simulink model " PV_PEM_reconfigurable_battery"  (R2026a)
settings: Solver=VariableStepAuto  StopTime=sim_t
undefined symbols (not defined in the file or in its folder): Active_Area, Bi_L, N, Q_batt, Ra_stack, Rc_stack, Rint_stack, sample_output_time, SOC_max, SOC_min, THR_75_down, THR_75_up, THR_97_down, THR_97_up, Ts, V_ref_battery, Vint_stack
libraries: fl_lib x30, nesl_utility x22, ee_lib x5, simulink x4, batteryecm_lib x1, slpidlib x1
settings Model: Creator=hanna  LastModifiedBy=Diamantis
settings SimscapeCC: SimscapeNominalValues="[{\"value\":\"1\",\"unit\":\"A\"},{\"value\":\"1\",\"unit\":\"bar\"},{\"value\":\"1\",\"unit\":\"cm^2\"},{\"value\":\"1\",\"unit\":\"cm^3/s\"},{\"value\":\"1\",\"unit\":\"kJ/kg\"},{\"value\":\"1\",\"unit\":\"kW\"},{\"value\":\"1\",\"unit\":\"l\"},{\"value\":\"1\",\"unit\":\"N\"},{\"value\":\"1\",\"unit\":\"N*m\"},{\"value\":\"1\",\"unit\":\"V\"}]"  SimscapeLogType=none  SimscapeLogDataHistory=5000.0

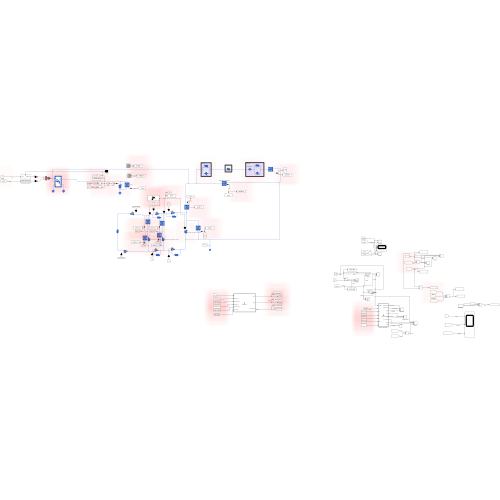
[thumbnail: Simulink's stored preview of the top-level diagram]
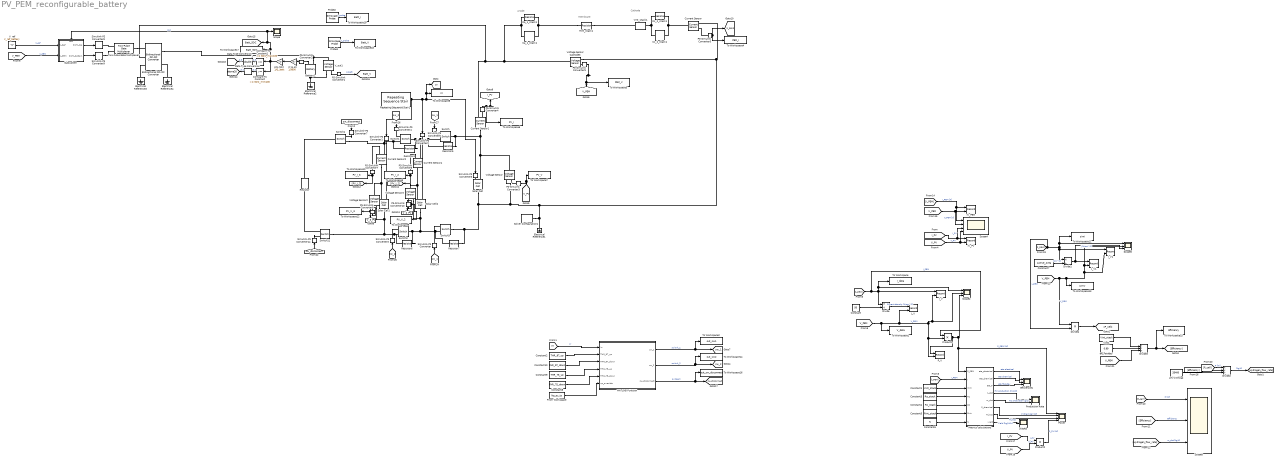
== system  PV_PEM_reconfigurable_battery ==
  note: Membrane
  note: Cathode
  note: Anode
  Battery1 : batteryecm_lib/Battery  Vnom=V_batt_nom V  prm_dir=simscape.enum.battery.prm_dir.disabled  R1_dis=0.05 Ohm  R1_ch=0.05 Ohm  R1=0.01 Ohm  prm_AH=simscape.enum.battery.prm_AH.finite  AH=Q_batt A*hr  V1=11.5 V  AH1=Q_batt*(SOC_min/100) A*hr  prm_R2=simscape.enum.battery.prm_R2.disabled  R2=2000 Ohm  Tmeas=298.15 K  charge_measurement_port=simscape.enum.battery.enable.yes  prm_dyn=simscape.enum.battery.prm_dyn.off  Rp1=0.005 Ohm  tau1=30 s  Rp2=0.005 Ohm  tau2=30 s  Rp3=0.005 Ohm  tau3=30 s  Rp4=0.005 Ohm  tau4=30 s  Rp5=0.005 Ohm  tau5=30 s  prm_fade=simscape.enum.battery.prm_fade.disabled  N_fade=100  AH_fade=45 A*hr  R1_fade=2.02 Ohm  R1_ch_fade=2.02 Ohm  V1_fade=10.35 V  prm_age=simscape.enum.battery.prm_age.disabled  prm_age_OCV=simscape.enum.battery.prm_age_OCV.OCV  OCV_age=0.9  SOC_age=60  Tmeas_age=298.15 K  delta_time_age_vec=[0] d  temperature_age_vec=[273] K  OCV_scaling_age=2.2134e6  OCV_offset_age=1.632e6  temp_exp_age=0.515833569 V  t_exp_age=0.75  Vnom_T2=12 V  R1_T2=2.2 Ohm  R1_T2_dis=2.2 Ohm  R1_T2_ch=2.2 Ohm  V1_T2=11.4 V  R2_T2=2200 Ohm  Rp1_T2=0.005 Ohm  tau1_T2=30 s  Rp2_T2=0.005 Ohm  tau2_T2=30 s  Rp3_T2=0.005 Ohm  tau3_T2=30 s  Rp4_T2=0.005 Ohm  tau4_T2=30 s  Rp5_T2=0.005 Ohm  tau5_T2=30 s  Tmeas2=273.15 K  thermal_port=simscape.enum.thermaleffects.omit  thermal_mass=30000 J/K  i_specify=off  i_priority=None  i=0 A  i_nominal_specify=off  i_nominal_value=1  i_nominal_unit=A  v_specify=off  v_priority=None  v=0 V  v_nominal_specify=off  v_nominal_value=1  v_nominal_unit=V  charge_specify=on  charge_priority=High  charge=SOC_init A*hr  charge_nominal_specify=off  charge_nominal_value=1  charge_nominal_unit=A*hr  num_cycles_specify=off  num_cycles_priority=High  num_cycles=0  num_cycles_nominal_specify=off  num_cycles_nominal_value=1  num_cycles_nominal_unit=1  temperature_specify=off  temperature_priority=High  temperature=298.15 K  temperature_nominal_specify=off  temperature_nominal_value=1  temperature_nominal_unit=K
      settings: LibrarySourceBlock=batt_lib/Cells/Battery
  Bidirectional DC-DC Converter : ee_lib/Semiconductors & Converters/Converters/Bidirectional DC-DC Converter  fidelity_option=ee.enum.converters.fidelity.detailed  device_type=ee.enum.converters.switchingdevice.mosfet  Vf=0.8 V  Ron=0.001 Ohm  Rds=0.001 Ohm  Goff=1e-6 1/Ohm  Vth=2 V  Vgt=0.5 V  Vgt_off=-1 V  Ih=1 A  K=0  diode_param=ee.enum.converters.diode.nodynamics  diode_Vf=0.8 V  diode_Ron=0.001 Ohm  diode_Goff=1e-5 1/Ohm  diode_C=50 nF  diode_iRM=-5 A  diode_iF=50 A  diode_idot=-50 A/us  diode_trr_param=ee.enum.converters.diodetrr.trr_factor  diode_trr_factor=3  diode_trr=0.5 us  diode_Qrr=1500 s*uA  L=Bi_L H  Rl=0 Ohm  C1=Bi_C1 F  C2=Bi_C2 F  R1=Bi_R1 Ohm  R2=Bi_R2 Ohm  snubber_type=ee.enum.converters.snubber.exclude  Cs=1e-7 F  Rs=0.1 Ohm  iL_specify=off  iL_priority=High  iL=0 A  iL_nominal_specify=off  iL_nominal_value=1  iL_nominal_unit=A  vc1_specify=off  vc1_priority=High  vc1=0 V  vc1_nominal_specify=off  vc1_nominal_value=1  vc1_nominal_unit=V  vc2_specify=off  vc2_priority=High  vc2=0 V  vc2_nominal_specify=off  vc2_nominal_value=1  vc2_nominal_unit=V  device_type_hv=ee.enum.converters.switchingdevice.ideal  Vf_hv=0.8 V  Ron_hv=0.001 Ohm  Rds_hv=0.001 Ohm  Goff_hv=1e-5 1/Ohm  Vth_hv=0.5 V  Vgt_hv=0.5 V  Vgt_off_hv=-1 V  Ih_hv=1 A  device_type_lv=ee.enum.converters.switchingdevice.ideal  Vf_lv=0.8 V  Ron_lv=0.001 Ohm  Rds_lv=0.001 Ohm  Goff_lv=1e-5 1/Ohm  Vth_lv=0.5 V  Vgt_lv=0.5 V  Vgt_off_lv=-1 V  Ih_lv=1 A  T_L1=0.03 H  T_L2=0.03 H  T_k=0.9  snubber_type_hv=ee.enum.converters.snubber.exclude  Cs_hv=1e-7 F  Rs_hv=0.1 Ohm  snubber_type_lv=ee.enum.converters.snubber.exclude  Cs_lv=1e-7 F  Rs_lv=0.1 Ohm  iL1_specify=off  iL1_priority=High  iL1=0 A  iL1_nominal_specify=off  iL1_nominal_value=1  iL1_nominal_unit=A  iL2_specify=off  iL2_priority=High  iL2=0 A  iL2_nominal_specify=off  iL2_nominal_value=1  iL2_nominal_unit=A  hysteresisCurrent=0.01 A
  C to Ah : Gain  Gain=1/3600
  Ca_1_stack1 : fl_lib/Electrical/Electrical Elements/Capacitor  c=Ca_stack F  r=1e-6 Ohm  g=0 1/Ohm  i_specify=off  i_priority=None  i=0 A  i_nominal_specify=off  i_nominal_value=1  i_nominal_unit=A  v_specify=off  v_priority=None  v=0 V  v_nominal_specify=off  v_nominal_value=1  v_nominal_unit=V  vc_specify=off  vc_priority=High  vc=0 V  vc_nominal_specify=off  vc_nominal_value=1  vc_nominal_unit=V
  Cc_2_stack1 : fl_lib/Electrical/Electrical Elements/Capacitor  c=Cc_stack F  r=1e-6 Ohm  g=0 1/Ohm  i_specify=off  i_priority=None  i=0 A  i_nominal_specify=off  i_nominal_value=1  i_nominal_unit=A  v_specify=off  v_priority=None  v=0 V  v_nominal_specify=off  v_nominal_value=1  v_nominal_unit=V  vc_specify=off  vc_priority=High  vc=0 V  vc_nominal_specify=off  vc_nominal_value=1  vc_nominal_unit=V
  Compare To Constant : simulink/Logic and Bit Operations/Compare To Constant  relop=>=  const=SOC_min/100  OutDataTypeStr=boolean
  Compare To Constant1 : simulink/Logic and Bit Operations/Compare To Constant  relop=<=  const=SOC_max/100  OutDataTypeStr=boolean
  Constant : Constant  Value=50
  Constant1 : Constant  Value=Vint_stack
  Constant10 : Constant  Value=THR_97_down
  Constant2 : Constant  Value=THR_97_up
  Constant3 : Constant  Value=Ra_stack
  Constant4 : Constant  Value=Rc_stack
  Constant5 : Constant  Value=Rint_stack
  Constant6 : Constant  Value=N
  Constant7 : Constant  Value=Active_Area
  Constant8 : Constant  Value=THR_75_down
  Constant9 : Constant  Value=THR_75_up
  Current Sensor{,1..2,4} (4 alike) : fl_lib/Electrical/Electrical Sensors/Current Sensor
  Data Type Conversion : DataTypeConversion  OutDataTypeStr=double  SaturateOnIntegerOverflow=off  RndMeth=Floor
  Data Type Conversion1 : DataTypeConversion  OutDataTypeStr=double  SaturateOnIntegerOverflow=off  RndMeth=Floor
  Divide : Product  Inputs=*/
  Divide1 : Product  Inputs=*/
  Divide2 : Product  Inputs=**/
  Divide3 : Product  Inputs=**/
  Divide4 : Product  Inputs=**
  Efficiencies : Scope  NumInputPorts=3
      settings: ActiveDisplayYMinimum=-1  ActiveDisplayYMaximum=1  DataLoggingMaxPoints=520000  DataLoggingVariableName=ScopeData5
  Electrical Reference{1..4} (4 alike) : fl_lib/Electrical/Electrical Elements/Electrical Reference
  From Workspace : FromWorkspace  VariableName=Np_py_ts
  IV_PEM : Record  NumPorts=2.0  FileSettingsInternal="{\"entries\":[{\"content\":{\"excelSettings\":{\"content\":{},\"type\":\"Streamout.ExcelSettings\"},\"parquetSettings\":{\"content\":{},\"type\":\"Streamout.ParquetSettings\"}},\"type\":\"Streamout.FileSettingStorage\",\"uuid\":\"\"}],\"packageUris\":[\"http:\\/\\/schema.mathworks.com\\/mf0\\/streamout_blocks\\/R2020a\"],\"version\":\"1.0\"}"  FrameSettings=[0, 0]  Layout=[1 1]  SignalsInternal="{\"entries\":[{\"content\":{\"signals\":[{\"content\":{\"blockPath\":[],\"dimensions\":[1],\"domain\":\"\",\"lineColor\":\"#edb120\",\"lineWidth\":2,\"port\":1,\"signalID\":1,\"signalName\":\"I_PEM [A]\"},\"type\":\"RecordBlkView.Signal\",\"uuid\":\"\"},{\"content\":{\"blockPath\":[],\"dimensions\":[1],\"domain\":\"\",\"lineColor\":\"#7e2f8e\",\"lineWidth\":2,\"port\":2,\"signalID\":2,\"signalName\":\"V_PEM [V]\"},\"type\":\"RecordBlkView.Signal\",\"uuid\":\"\"}]},\"type\":\"RecordBlkView.InputSignals\",\"uuid\":\"\"}],\"packageUris\":[\"http:\\/\\/schema.mathworks.com\\/mf0\\/streamout_blocks\\/R2020a\"],\"version\":\"1.0\"}"  VisualizationBindings="{\"xyplotplugin\":{\"info\":[{\"series\":[],\"subplotID\":1}]}}"  CompatibilityTag=XY
  IV_PV : Record  NumPorts=2.0  FileSettingsInternal="{\"entries\":[{\"content\":{\"excelSettings\":{\"content\":{},\"type\":\"Streamout.ExcelSettings\"},\"parquetSettings\":{\"content\":{},\"type\":\"Streamout.ParquetSettings\"}},\"type\":\"Streamout.FileSettingStorage\",\"uuid\":\"\"}],\"packageUris\":[\"http:\\/\\/schema.mathworks.com\\/mf0\\/streamout_blocks\\/R2020a\"],\"version\":\"1.0\"}"  FrameSettings=[0, 0]  Layout=[1 1]  SignalsInternal="{\"entries\":[{\"content\":{\"signals\":[{\"content\":{\"blockPath\":[],\"dimensions\":[1],\"domain\":\"\",\"lineColor\":\"#a2142f\",\"plots\":[ 1 ],\"port\":1,\"signalID\":1,\"signalName\":\"I_PV\"},\"type\":\"RecordBlkView.Signal\",\"uuid\":\"\"},{\"content\":{\"blockPath\":[],\"dimensions\":[1],\"domain\":\"\",\"lineColor\":\"#139fff\",\"plots\":[ 1 ],\"port\":2,\"signalID\":2,\"signalName\":\"V_PV\"},\"type\":\"RecordBlkView.Signal\",\"uuid\":\"\"}]},\"type\":\"RecordBlkView.InputSignals\",\"uuid\":\"\"}],\"packageUris\":[\"http:\\/\\/schema.mathworks.com\\/mf0\\/streamout_blocks\\/R2020a\"],\"version\":\"1.0\"}"  VisualizationBindings="{\"xyplotplugin\":{\"info\":[{\"series\":[{\"bindingParametersList\":[{\"parameter\":\"X-Axis\",\"signalID\":1,\"signalName\":\"I_PV\"},{\"parameter\":\"Y-Axis\",\"signalID\":2,\"signalName\":\"V_PV\"}],\"seriesID\":0}],\"subplotID\":1}]}}"  CompatibilityTag=XY
  I_V : Record  NumPorts=2.0  FileSettingsInternal="{\"entries\":[{\"content\":{\"excelSettings\":{\"content\":{},\"type\":\"Streamout.ExcelSettings\"},\"parquetSettings\":{\"content\":{},\"type\":\"Streamout.ParquetSettings\"}},\"type\":\"Streamout.FileSettingStorage\",\"uuid\":\"\"}],\"packageUris\":[\"http:\\/\\/schema.mathworks.com\\/mf0\\/streamout_blocks\\/R2020a\"],\"version\":\"1.0\"}"  FrameSettings=[0, 0]  Layout=[1 1]  SignalsInternal="{\"entries\":[{\"content\":{\"signals\":[{\"content\":{\"blockPath\":[],\"dimensions\":[1],\"domain\":\"\",\"lineColor\":\"#a2142f\",\"lineWidth\":2,\"port\":1,\"signalID\":1,\"signalName\":\"I_PEM\"},\"type\":\"RecordBlkView.Signal\",\"uuid\":\"\"},{\"content\":{\"blockPath\":[],\"dimensions\":[1],\"domain\":\"\",\"lineColor\":\"#139fff\",\"lineWidth\":2,\"port\":2,\"signalID\":2,\"signalName\":\"V_PEM\"},\"type\":\"RecordBlkView.Signal\",\"uuid\":\"\"}]},\"type\":\"RecordBlkView.InputSignals\",\"uuid\":\"\"}],\"packageUris\":[\"http:\\/\\/schema.mathworks.com\\/mf0\\/streamout_blocks\\/R2020a\"],\"version\":\"1.0\"}"  VisualizationBindings="{\"xyplotplugin\":{\"info\":[{\"series\":[],\"subplotID\":1}]}}"  CompatibilityTag=XY
  I_V1 : Record  NumPorts=2.0  FileSettingsInternal="{\"entries\":[{\"content\":{\"excelSettings\":{\"content\":{},\"type\":\"Streamout.ExcelSettings\"},\"parquetSettings\":{\"content\":{},\"type\":\"Streamout.ParquetSettings\"}},\"type\":\"Streamout.FileSettingStorage\",\"uuid\":\"\"}],\"packageUris\":[\"http:\\/\\/schema.mathworks.com\\/mf0\\/streamout_blocks\\/R2020a\"],\"version\":\"1.0\"}"  FrameSettings=[0, 0]  Layout=[1 1]  SignalsInternal="{\"entries\":[{\"content\":{\"signals\":[{\"content\":{\"blockPath\":[],\"dimensions\":[1],\"domain\":\"\",\"lineColor\":\"#ff6929\",\"lineWidth\":2,\"port\":1,\"signalID\":1,\"signalName\":\"I_PEM\"},\"type\":\"RecordBlkView.Signal\",\"uuid\":\"\"},{\"content\":{\"blockPath\":[],\"dimensions\":[1],\"domain\":\"\",\"lineColor\":\"#b746ff\",\"lineWidth\":2,\"port\":2,\"signalID\":2,\"signalName\":\"V_PEM\"},\"type\":\"RecordBlkView.Signal\",\"uuid\":\"\"}]},\"type\":\"RecordBlkView.InputSignals\",\"uuid\":\"\"}],\"packageUris\":[\"http:\\/\\/schema.mathworks.com\\/mf0\\/streamout_blocks\\/R2020a\"],\"version\":\"1.0\"}"  VisualizationBindings="{\"xyplotplugin\":{\"info\":[{\"series\":[],\"subplotID\":1}]}}"  CompatibilityTag=XY
  J_V : Record  NumPorts=2.0  FileSettingsInternal="{\"entries\":[{\"content\":{\"excelSettings\":{\"content\":{},\"type\":\"Streamout.ExcelSettings\"},\"parquetSettings\":{\"content\":{},\"type\":\"Streamout.ParquetSettings\"}},\"type\":\"Streamout.FileSettingStorage\",\"uuid\":\"\"}],\"packageUris\":[\"http:\\/\\/schema.mathworks.com\\/mf0\\/streamout_blocks\\/R2020a\"],\"version\":\"1.0\"}"  FrameSettings=[0, 0]  Layout=[1 1]  SignalsInternal="{\"entries\":[{\"content\":{\"signals\":[{\"content\":{\"blockPath\":[],\"dimensions\":[1],\"domain\":\"\",\"lineColor\":\"#64d413\",\"lineWidth\":2,\"port\":1,\"signalID\":1,\"signalName\":\"Current density [A\\/cm^2]\"},\"type\":\"RecordBlkView.Signal\",\"uuid\":\"\"},{\"content\":{\"blockPath\":[],\"dimensions\":[1],\"domain\":\"\",\"lineColor\":\"#ff13a6\",\"lineWidth\":2,\"port\":2,\"signalID\":2,\"signalName\":\"V_PEM\"},\"type\":\"RecordBlkView.Signal\",\"uuid\":\"\"}]},\"type\":\"RecordBlkView.InputSignals\",\"uuid\":\"\"}],\"packageUris\":[\"http:\\/\\/schema.mathworks.com\\/mf0\\/streamout_blocks\\/R2020a\"],\"version\":\"1.0\"}"  VisualizationBindings="{\"xyplotplugin\":{\"info\":[{\"series\":[],\"subplotID\":1}]}}"  CompatibilityTag=XY
  J_V1 : Record  NumPorts=2.0  FileSettingsInternal="{\"entries\":[{\"content\":{\"excelSettings\":{\"content\":{},\"type\":\"Streamout.ExcelSettings\"},\"parquetSettings\":{\"content\":{},\"type\":\"Streamout.ParquetSettings\"}},\"type\":\"Streamout.FileSettingStorage\",\"uuid\":\"\"}],\"packageUris\":[\"http:\\/\\/schema.mathworks.com\\/mf0\\/streamout_blocks\\/R2020a\"],\"version\":\"1.0\"}"  FrameSettings=[0, 0]  Layout=[1 1]  SignalsInternal="{\"entries\":[{\"content\":{\"signals\":[{\"content\":{\"blockPath\":[],\"dimensions\":[1],\"domain\":\"\",\"lineColor\":\"#fe330a\",\"lineWidth\":2,\"port\":1,\"signalID\":1,\"signalName\":\"J [A\\/cm^2]\"},\"type\":\"RecordBlkView.Signal\",\"uuid\":\"\"},{\"content\":{\"blockPath\":[],\"dimensions\":[1],\"domain\":\"\",\"lineColor\":\"#22b573\",\"lineWidth\":2,\"port\":2,\"signalID\":2,\"signalName\":\"V_PEM\"},\"type\":\"RecordBlkView.Signal\",\"uuid\":\"\"}]},\"type\":\"RecordBlkView.InputSignals\",\"uuid\":\"\"}],\"packageUris\":[\"http:\\/\\/schema.mathworks.com\\/mf0\\/streamout_blocks\\/R2020a\"],\"version\":\"1.0\"}"  VisualizationBindings="{\"xyplotplugin\":{\"info\":[{\"series\":[],\"subplotID\":1}]}}"  CompatibilityTag=XY
  LHV [Wh/kg] : Constant  Value=33400
  MATLAB Function : MATLAB Function  TreatAsAtomicUnit=on
  Metrics calculations : MATLAB Function  TreatAsAtomicUnit=on
  PS-Simulink Converter{1..2,5..7,9} (6 alike) : nesl_utility/PS-Simulink Converter  PhysicalDomain=network_engine_domain  SubClassName=ps_output  LeftPortType=input  RightPortType=output  PseudoPeriodic=off  Frequencies=[]  VectorFormat=inherit  Unit=inherit  AffineConversion=off
  PS-Simulink Converter10 : nesl_utility/PS-Simulink Converter  PhysicalDomain=network_engine_domain  SubClassName=ps_output  LeftPortType=input  RightPortType=output  PseudoPeriodic=off  Frequencies=[]  VectorFormat=1-D array  Unit=V  AffineConversion=off
  PS-Simulink Converter3 : nesl_utility/PS-Simulink Converter  PhysicalDomain=network_engine_domain  SubClassName=ps_output  LeftPortType=input  RightPortType=output  PseudoPeriodic=off  Frequencies=[]  VectorFormat=1-D array  Unit=V  AffineConversion=off
  PS-Simulink Converter4 : nesl_utility/PS-Simulink Converter  PhysicalDomain=network_engine_domain  SubClassName=ps_output  LeftPortType=input  RightPortType=output  PseudoPeriodic=off  Frequencies=[]  VectorFormat=1-D array  Unit=A  AffineConversion=off
  PS-Simulink Converter8 : nesl_utility/PS-Simulink Converter  PhysicalDomain=network_engine_domain  SubClassName=ps_output  LeftPortType=input  RightPortType=output  PseudoPeriodic=off  Frequencies=[]  VectorFormat=1-D array  Unit=V  AffineConversion=off
  P_V : Record  NumPorts=2.0  FileSettingsInternal="{\"entries\":[{\"content\":{\"excelSettings\":{\"content\":{},\"type\":\"Streamout.ExcelSettings\"},\"parquetSettings\":{\"content\":{},\"type\":\"Streamout.ParquetSettings\"}},\"type\":\"Streamout.FileSettingStorage\",\"uuid\":\"\"}],\"packageUris\":[\"http:\\/\\/schema.mathworks.com\\/mf0\\/streamout_blocks\\/R2020a\"],\"version\":\"1.0\"}"  FrameSettings=[0, 0]  Layout=[1 1]  SignalsInternal="{\"entries\":[{\"content\":{\"signals\":[{\"content\":{\"blockPath\":[],\"dimensions\":[1],\"domain\":\"\",\"lineColor\":\"#0072bd\",\"lineWidth\":2,\"port\":1,\"signalID\":1,\"signalName\":\"P_PEM [W]\"},\"type\":\"RecordBlkView.Signal\",\"uuid\":\"\"},{\"content\":{\"blockPath\":[],\"dimensions\":[1],\"domain\":\"\",\"lineColor\":\"#d95319\",\"lineWidth\":2,\"port\":2,\"signalID\":2,\"signalName\":\"V_PEM\"},\"type\":\"RecordBlkView.Signal\",\"uuid\":\"\"}]},\"type\":\"RecordBlkView.InputSignals\",\"uuid\":\"\"}],\"packageUris\":[\"http:\\/\\/schema.mathworks.com\\/mf0\\/streamout_blocks\\/R2020a\"],\"version\":\"1.0\"}"  VisualizationBindings="{\"xyplotplugin\":{\"info\":[{\"series\":[],\"subplotID\":1}]}}"  CompatibilityTag=XY
  Power : Scope  NumInputPorts=4
      settings: ActiveDisplayYMinimum=-1  ActiveDisplayYMaximum=1  DataLoggingMaxPoints=520000  DataLoggingVariableName=ScopeData6
  Probe1 : SimscapeProbe  BoundBlock=1128  Variables="{\"i\":{\"Probing\":\"OFF\"},\"n.v\":{\"Probing\":\"OFF\"},\"p.v\":{\"Probing\":\"OFF\"},\"v\":{\"Probing\":\"ON\"}}"
  Probe2 : SimscapeProbe  BoundBlock=1128  Variables="{\"i\":{\"Probing\":\"ON\"}}"
  Product1 : Product
  Product2 : Product
  Production Rate : Scope  NumInputPorts=2
      settings: ActiveDisplayYMinimum=-6.6507662971533038E-5  ActiveDisplayYMaximum=0.00059856896673107221  DataLoggingMaxPoints=520000  DataLoggingVariableName=ScopeData7
  Ra_1_stack1 : fl_lib/Electrical/Electrical Elements/Resistor  R=Ra_stack Ohm  i_specify=off  i_priority=None  i=0 A  i_nominal_specify=off  i_nominal_value=1  i_nominal_unit=A  v_specify=off  v_priority=None  v=0 V  v_nominal_specify=off  v_nominal_value=1  v_nominal_unit=V
  Rc_2_stack1 : fl_lib/Electrical/Electrical Elements/Resistor  R=Rc_stack Ohm  i_specify=off  i_priority=None  i=0 A  i_nominal_specify=off  i_nominal_value=1  i_nominal_unit=A  v_specify=off  v_priority=None  v=0 V  v_nominal_specify=off  v_nominal_value=1  v_nominal_unit=V
  Repeating Sequence Stair1 : simulink/Sources/Repeating Sequence Stair  OutValues=Irr_stair_val  tsamp=Irr_stair_tsamp  OutMin=[]  OutMax=[]  OutDataTypeStr=double  OutputDataTypeScalingMode=double  OutDataType=fixdt(0,8)  ConRadixGroup=Best Precision: Vector-wise  OutScaling=2^-12
  Resistor : fl_lib/Electrical/Electrical Elements/Resistor  R=1 Ohm  i_specify=off  i_priority=None  i=0 A  i_nominal_specify=off  i_nominal_value=1  i_nominal_unit=A  v_specify=off  v_priority=None  v=0 V  v_nominal_specify=off  v_nominal_value=1  v_nominal_unit=V
  Resistor{4..7} (4 alike) : fl_lib/Electrical/Electrical Elements/Resistor  R=1e6 Ohm  i_specify=off  i_priority=None  i=0 A  i_nominal_specify=off  i_nominal_value=1  i_nominal_unit=A  v_specify=off  v_priority=None  v=0 V  v_nominal_specify=off  v_nominal_value=1  v_nominal_unit=V
  Rint_stack1 : fl_lib/Electrical/Electrical Elements/Resistor  R=Rint_stack Ohm  i_specify=off  i_priority=None  i=0 A  i_nominal_specify=off  i_nominal_value=1  i_nominal_unit=A  v_specify=off  v_priority=None  v=0 V  v_nominal_specify=off  v_nominal_value=1  v_nominal_unit=V
  Scope : Scope
      settings: ActiveDisplayYMinimum=0.599999044089406  ActiveDisplayYMaximum=0.60000010621228816  DataLoggingVariableName=ScopeData4
  Scope2 : Scope  NumInputPorts=3
      settings: ActiveDisplayYMinimum=-2.2100954998449684  ActiveDisplayYMaximum=19.79179103183268  DataLoggingMaxPoints=520000  DataLoggingVariableName=ScopeData2
  Scope3 : Scope
      settings: ActiveDisplayYMinimum=-1  ActiveDisplayYMaximum=1  DataLoggingMaxPoints=520000  DataLoggingVariableName=ScopeData3
  Scope4 : Scope  NumInputPorts=4
      settings: ActiveDisplayYMinimum=-6.1277884950416563  ActiveDisplayYMaximum=54.606123205001168  DataLoggingMaxPoints=520000  DataLoggingVariableName=ScopeData9
  Scope6 : Scope  NumInputPorts=3
      settings: ActiveDisplayYMinimum=2.1952046709351865  ActiveDisplayYMaximum=2.2345014292442293  DataLoggingMaxPoints=520000  DataLoggingVariableName=ScopeData10
  Scope8 : Scope  NumInputPorts=3
      settings: ActiveDisplayString=3  ActiveDisplayYMinimum=-0.0016083601949654486  ActiveDisplayYMaximum=0.014332465135728535  DataLoggingMaxPoints=520000
  Simulink-PS Converter{,1..7,14} (9 alike) : nesl_utility/Simulink-PS Converter  PhysicalDomain=network_engine_domain  SubClassName=ps_input  LeftPortType=input  RightPortType=output  PseudoPeriodic=off  Frequencies=[]  NoiseDistribution=none  NoiseParameters=[]  Unit=1  AffineConversion=off  FilteringAndDerivatives=provide  SimscapeFilterOrder=1  InputFilterTimeConstant=0.001  UdotUserProvided=0
  Simulink-PS Converter8 : nesl_utility/Simulink-PS Converter  PhysicalDomain=network_engine_domain  SubClassName=ps_input  LeftPortType=input  RightPortType=output  PseudoPeriodic=off  Frequencies=[]  NoiseDistribution=none  NoiseParameters=[]  Unit=1  AffineConversion=off  FilteringAndDerivatives=provide  SimscapeFilterOrder=1  InputFilterTimeConstant=1e-7  UdotUserProvided=0
  Simulink-PS Converter9 : nesl_utility/Simulink-PS Converter  PhysicalDomain=network_engine_domain  SubClassName=ps_input  LeftPortType=input  RightPortType=output  PseudoPeriodic=off  Frequencies=[]  NoiseDistribution=none  NoiseParameters=[]  Unit=1  AffineConversion=off  FilteringAndDerivatives=provide  SimscapeFilterOrder=1  InputFilterTimeConstant=1e-7  UdotUserProvided=0
  Solar Cell : ee_lib/Sources/Solar Cell  PartSpecification="{\"CollectionId\":\"SimscapeElectrical\",\"CollectionVersion\":\"1.0.0\",\"DatasetId\":\"Amerisolar|AS_6M30_HC_320W|simscape.electrical.solarCell\",\"DisplayName\":\"Amerisolar:AS_6M30_HC_320W\"}"  prm=3  Isc=10.14 % Datasheet derived A  Voc=0.67 % Datasheet derived V  Is=3.24823447983853e-07 % Datasheet derived A  Is2=9.37081970792037e-10 % Datasheet derived A  Iph=10.140005507508 % Datasheet derived A  Ir0=1000 % Datasheet derived W/m^2  ec=1.51118472243322 % Datasheet derived  N2=2.60259908345858 % Datasheet derived  Rs=1.94548269975201e-05 % Datasheet derived Ohm  Rp=682.95993142779 % Datasheet derived Ohm  N_series=Ns_cell % Datasheet derived  N_parallel=Np_cell_base % Datasheet derived  TIPH1=0.000499942933005141 % Datasheet derived 1/K  EG=1.12 % Datasheet derived eV  TXIS1=4.23641510120988 % Datasheet derived  TXIS2=16.2689137700667 % Datasheet derived  TRS1=0.243341028305912 % Datasheet derived  TRP1=0 % Parameter not set  Tmeas=25 % Datasheet derived degC  TFIXED=25 % Datasheet derived degC  thermal_mass=100 % Parameter not set J/K  initial_temperature=25 degC
      settings: AttributesFormatString=Amerisolar:AS_6M30_HC_320W
  Solar Cell1 : ee_lib/Sources/Solar Cell  PartSpecification="{\"CollectionId\":\"SimscapeElectrical\",\"CollectionVersion\":\"1.0.0\",\"DatasetId\":\"Amerisolar|AS_6M30_HC_320W|simscape.electrical.solarCell\",\"DisplayName\":\"Amerisolar:AS_6M30_HC_320W\"}"  prm=3  Isc=10.14 % Datasheet derived A  Voc=0.67 % Datasheet derived V  Is=3.24823447983853e-07 % Datasheet derived A  Is2=9.37081970792037e-10 % Datasheet derived A  Iph=10.140005507508 % Datasheet derived A  Ir0=1000 % Datasheet derived W/m^2  ec=1.51118472243322 % Datasheet derived  N2=2.60259908345858 % Datasheet derived  Rs=1.94548269975201e-05 % Datasheet derived Ohm  Rp=682.95993142779 % Datasheet derived Ohm  N_series=Ns_cell % Datasheet derived  N_parallel=Np_cell_add_2 % Datasheet derived  TIPH1=0.000499942933005141 % Datasheet derived 1/K  EG=1.12 % Datasheet derived eV  TXIS1=4.23641510120988 % Datasheet derived  TXIS2=16.2689137700667 % Datasheet derived  TRS1=0.243341028305912 % Datasheet derived  TRP1=0 % Parameter not set  Tmeas=25 % Datasheet derived degC  TFIXED=25 % Datasheet derived degC  thermal_mass=100 % Parameter not set J/K  initial_temperature=25 degC
      settings: AttributesFormatString=Amerisolar:AS_6M30_HC_320W
  Solar Cell2 : ee_lib/Sources/Solar Cell  PartSpecification="{\"CollectionId\":\"SimscapeElectrical\",\"CollectionVersion\":\"1.0.0\",\"DatasetId\":\"Amerisolar|AS_6M30_HC_320W|simscape.electrical.solarCell\",\"DisplayName\":\"Amerisolar:AS_6M30_HC_320W\"}"  prm=3  Isc=10.14 % Datasheet derived A  Voc=0.67 % Datasheet derived V  Is=3.24823447983853e-07 % Datasheet derived A  Is2=9.37081970792037e-10 % Datasheet derived A  Iph=10.140005507508 % Datasheet derived A  Ir0=1000 % Datasheet derived W/m^2  ec=1.51118472243322 % Datasheet derived  N2=2.60259908345858 % Datasheet derived  Rs=1.94548269975201e-05 % Datasheet derived Ohm  Rp=682.95993142779 % Datasheet derived Ohm  N_series=Ns_cell % Datasheet derived  N_parallel=Np_cell_add_1 % Datasheet derived  TIPH1=0.000499942933005141 % Datasheet derived 1/K  EG=1.12 % Datasheet derived eV  TXIS1=4.23641510120988 % Datasheet derived  TXIS2=16.2689137700667 % Datasheet derived  TRS1=0.243341028305912 % Datasheet derived  TRP1=0 % Parameter not set  Tmeas=25 % Datasheet derived degC  TFIXED=25 % Datasheet derived degC  thermal_mass=100 % Parameter not set J/K  initial_temperature=25 degC
      settings: AttributesFormatString=Amerisolar:AS_6M30_HC_320W
  Solver Configuration1 : nesl_utility/Solver Configuration  PhysicalDomain=network_engine_domain  SubClassName=solver  LeftPortType=input  RightPortType=generic  Tones=[]  Harmonics=[]  SimulateNoise=off  Profile=off  UseLocalSampling=off  EnableSwitchedLinearOptims=on  FrequencyDomain=off  UseCCode=off  RelTol=0.001  AbsTol=0.001  MinStep=1e-09  ToWorkspace=off  RevertToSquareIcSolve=off  NumHomotopyIterations=100  PhasorMode=off  PhasorModeNumHarmonics=1  ConsistencySolver=NEWTON_XTOL_AFTER_FTOL  CanonicalOrdering=UNORDERED  OptimizeIntermediates=UNOPTIMIZED  IndexReductionMethod=DerivativeReplacement  DoDC=off  ResidualTolerance=1e-09  ConsistencyTolSource=GLOBAL  ConsistencyAbsTol=0.001  ConsistencyRelTol=0.001  ConsistencyTolFactor=0.001  UseLocalSolver=off  LocalSolverChoice=NE_BACKWARD_EULER_ADVANCER  ResolveIndetEquations=on  FunctionEvalNumThread=1  LocalSolverSampleTime=0.001  DoFixedCost=off  MaxNonlinIter=3  MaxModeIter=2  ComputeImpulses=off  ImpulseIterations=2  LinearAlgebra=auto  LinearAlgebraNumThread=0  EquationFormulation=NE_TIME_EF  DelaysMemoryBudget=1024  AutomaticFiltering=on  FilteringTimeConstant=0.001  PartitionStorageMethod=AS_NEEDED  PartitionMemoryBudget=1024  PartitionMethod=ROBUST  MultibodyUseLocalSolver=off  MultibodyLocalSolverChoice=ODE1  MultibodyLocalSolverSampleTime=0.001
  Subsystem : Subsystem
      settings: PortSchema="{\"entries\":[{\"content\":{\"sides\":[{\"content\":{\"connectorIds\":[\"In1\",\"In2\"]},\"type\":\"ConnectorPlacement.EquallySpacedRectSide\",\"uuid\":\"4e9ec41c-bdf9-454a-9c62-b3d400a7e8a5\"},{\"content\":{\"connectorIds\":[\"Out1\",\"Out2\"],\"side\":\"RIGHT\"},\"type\":\"ConnectorPlacement.EquallySpacedRectSide\",\"uuid\":\"9c7ad0fb-9491-4539-a93e-b9f6c9148e2a\"},{\"content\":{\"connectorIds\":[\"In3\"],\"side\":\"TOP\"},\"type\":\"ConnectorPlacement.EquallySpacedRectSide\",\"uuid\":\"b08aae61-0a78-4c70-83b8-04326ad74e93\"}]},\"type\":\"ConnectorPlacement.EquallySpacedConnector\",\"uuid\":\"604710b3-7757-4fb6-916a-2f806a8ce5d4\"}],\"packageUris\":[\"http://schema.mathworks.com/mf0/Connector/R2020b\"],\"version\":\"1.0\"}"
  Switch{,1..4,11} (6 alike) : fl_lib/Electrical/Electrical Elements/Switch  R_closed=0.01 Ohm  G_open=1e-8 1/Ohm  Threshold=0.5  i_specify=off  i_priority=None  i=0 A  i_nominal_specify=off  i_nominal_value=1  i_nominal_unit=A  v_specify=off  v_priority=None  v=0 V  v_nominal_specify=off  v_nominal_value=1  v_nominal_unit=V
  To Workspace : ToWorkspace  VariableName=I_data  SaveFormat=Timeseries  SampleTime=-1
  To Workspace1 : ToWorkspace  VariableName=V_data  SaveFormat=Timeseries  SampleTime=-1
  To Workspace10 : ToWorkspace  VariableName=PV_I_3  SaveFormat=Timeseries  SampleTime=sample_output_time
  To Workspace11 : ToWorkspace  VariableName=simI  SaveFormat=Timeseries  SampleTime=0.1
  To Workspace12 : ToWorkspace  VariableName=PV_V_3  SaveFormat=Timeseries  SampleTime=sample_output_time
  To Workspace13 : ToWorkspace  VariableName=simV  SaveFormat=Timeseries  SampleTime=0.1
  To Workspace14 : ToWorkspace  VariableName=out_sw2  SaveFormat=Timeseries  SampleTime=sample_output_time
  To Workspace15 : ToWorkspace  VariableName=Efficiency  SaveFormat=Timeseries  SampleTime=-1
  To Workspace16 : ToWorkspace  VariableName=out_sw_disconnect  SaveFormat=Timeseries  SampleTime=sample_output_time
  To Workspace17 : ToWorkspace  VariableName=Batt_SOC  SaveFormat=Timeseries  SampleTime=sample_output_time
  To Workspace18 : ToWorkspace  VariableName=Batt_V  SaveFormat=Timeseries  SampleTime=sample_output_time
  To Workspace19 : ToWorkspace  VariableName=Batt_I  SaveFormat=Timeseries  SampleTime=sample_output_time
  To Workspace2 : ToWorkspace  VariableName=out_sw1  SaveFormat=Timeseries  SampleTime=sample_output_time
  To Workspace3 : ToWorkspace  VariableName=PV_I_2  SaveFormat=Timeseries  SampleTime=sample_output_time
  To Workspace4 : ToWorkspace  VariableName=PEM_I  SaveFormat=Timeseries  SampleTime=sample_output_time
  To Workspace5 : ToWorkspace  VariableName=PEM_V  SaveFormat=Timeseries  SampleTime=sample_output_time
  To Workspace6 : ToWorkspace  VariableName=PV_I  SaveFormat=Timeseries  SampleTime=sample_output_time
  To Workspace7 : ToWorkspace  VariableName=PV_V  SaveFormat=Timeseries  SampleTime=sample_output_time
  To Workspace8 : ToWorkspace  VariableName=Irr  SaveFormat=Timeseries  SampleTime=sample_output_time
  To Workspace9 : ToWorkspace  VariableName=PV_V_2  SaveFormat=Timeseries  SampleTime=sample_output_time
  Two-Pulse Gate Multiplexer : ee_lib/Semiconductors & Converters/Converters/Two-Pulse Gate Multiplexer  port_option=ee.enum.controlport.ps
  V_out1 : fl_lib/Electrical/Electrical Sensors/Voltage Sensor
  V_ref : Constant  Value=V_ref_battery
  Vint1 : Constant  Value=Vint_stack
  Vint_stack1 : fl_lib/Electrical/Electrical Sources/DC Voltage Source  v0=Vint_stack V
  Voltage Sensor : fl_lib/Electrical/Electrical Sensors/Voltage Sensor
  Voltage Sensor Cathode3 : fl_lib/Electrical/Electrical Sensors/Voltage Sensor
  Voltage Sensor2 : fl_lib/Electrical/Electrical Sensors/Voltage Sensor
  Voltage Sensor3 : fl_lib/Electrical/Electrical Sensors/Voltage Sensor
  eff_Faraday : Constant  Value=0.99
  into SOC : Gain  Gain=1/Q_batt
  tag scope: Batt_SOC=global, Batt_V=global, I_PV=global, Irr=global, V_2_PV=global, V_3_PV=global, V_PEM=global, V_PV=global, above20=global, below90=global, sw_1=global, sw_2=global, sw_disconnect=global
  wires:
  PS-Simulink Converter9/1 -> To Workspace5/1, [V_PEM]
  PS-Simulink Converter4/1 -> To Workspace6/1, [I_PV]
  PS-Simulink Converter5/1 -> To Workspace4/1, [I_PEM]
  PS-Simulink Converter3/1 -> To Workspace7/1, [V_PV]
  PS-Simulink Converter7/1 -> [PV_I_3], To Workspace10/1
  Repeating Sequence Stair1/1 -> Simulink-PS Converter1/1, To Workspace8/1, [Irr], Simulink-PS Converter5/1, Simulink-PS Converter2/1
  [sw_1] -> Simulink-PS Converter/1
  [sw_2] -> Simulink-PS Converter3/1
  [sw_2] -> Simulink-PS Converter4/1
  [sw_1] -> Simulink-PS Converter6/1
  PS-Simulink Converter8/1 -> [V_3_PV], To Workspace12/1
  PS-Simulink Converter10/1 -> To Workspace9/1, [V_2_PV]
  PS-Simulink Converter6/1 -> [PV_I_2], To Workspace3/1
  [sw_disconnect] -> Simulink-PS Converter14/1
  [sw_disconnect] -> Simulink-PS Converter7/1
  Constant4/1 -> Metrics calculations/5(R2)
  [I_PEM] -> Scope6/1, To Workspace11/1, Divide1/1, I_V1/1, Divide4/2  "I_PEM"
  [V_PV] -> Scope4/4, IV_PV/2  "V_PV"
  Divide2/1 -> [Hydrogen_flow_rate]  "[kg/h]"
  [V_PEM] -> Scope4/2, IV_PEM/2  "V_PEM [V]"
  Metrics calculations/3(eta_F) -> Efficiencies/3  "eta Faraday"
  [V_PEM] -> I_V/2, Scope2/2, Product1/2, P_V/2, J_V/2, To Workspace1/1  "V_PEM"
  Divide4/1 -> [P_cell]
  [V_PV] -> Product2/2  "V_PV"
  [V_PEM] -> Divide3/3
  [P_cell] -> Scope8/1  "P [W]"
  Constant3/1 -> Metrics calculations/4(R1)
  Constant7/1 -> Divide1/2  "[cm^2]"
  LHV [Wh/kg]/1 -> Divide2/3
  Metrics calculations/1(eta_electrical) -> Efficiencies/1  "eta electrical"
  Product2/1 -> Power/4  "P_PV [W]"
  [Hydrogen_flow_rate] -> Scope8/3  "m_dot [kg/h]"
  Constant1/1 -> Metrics calculations/3(Vint)
  [I_PEM] -> Metrics calculations/2(I)  "I_PEM"
  Constant5/1 -> Metrics calculations/6(Rint)
  Metrics calculations/7(P_loss) -> Power/3  "P_loss"
  Product1/1 -> P_V/1, Metrics calculations/1(P_PEM), Power/1, Scope2/3  "P_PEM [W]"
  Vint1/1 -> Divide3/1
  [I_PEM] -> Scope4/1, IV_PEM/1  "I_PEM [A]"
  Divide3/1 -> To Workspace15/1, [Efficiency]
  eff_Faraday/1 -> Divide3/2
  [I_PV] -> Scope4/3, IV_PV/1  "I_PV"
  [Efficiency] -> Scope8/2  "Efficiency"
  Constant6/1 -> Metrics calculations/7(N)
  [I_PV] -> Product2/1  "I_PV"
  Divide/1 -> J_V/1  "Current density [A/cm^2]"
  Metrics calculations/4(n_dot) -> Production Rate/1  "H2 production [mol/s]"
  Metrics calculations/5(m_dot) -> Production Rate/2  "H2 production [g/s]"
  [P_cell] -> Divide2/1  "P [W]"
  Metrics calculations/2(eta_chemical) -> Efficiencies/2  "eta chemical"
  Constant/1 -> Divide/2
  [V_PEM] -> Divide4/1, To Workspace13/1, Scope6/2, J_V1/2, I_V1/2  "V_PEM"
  Divide1/1 -> Scope6/3, J_V1/1  "J [A/cm^2]"
  Metrics calculations/8(yield) -> Scope3/1  "Yield [kg/kWh]"
  [I_PEM] -> I_V/1, Divide/1, To Workspace/1, Scope2/1, Product1/1  "I_PEM"
  Metrics calculations/6(P_chemical) -> Power/2  "P Chemical [W]"
  [Efficiency] -> Divide2/2
  From Workspace/1 -> MATLAB Function/6(np_override)
  MATLAB Function/1(sw_1) -> To Workspace2/1, [sw_1]  "switxh_1"
  MATLAB Function/3(sw_disconnect) -> To Workspace16/1, [sw_disconnect]  "pv2pem"
  Constant2/1 -> MATLAB Function/2(THR_97_up)
  [Irr] -> MATLAB Function/1(irr)  "Irr"
  MATLAB Function/2(sw_2) -> To Workspace14/1, [sw_2]  "switxh_2"
  Constant9/1 -> MATLAB Function/4(THR_75_up)
  Constant8/1 -> MATLAB Function/5(THR_75_down)
  Constant10/1 -> MATLAB Function/3(THR_97_down)
  C to Ah/1 -> into SOC/1
  [V_PEM] -> Subsystem/2(V_PEM)  "V_PEM"
  Subsystem/1(PWM_top) -> Simulink-PS Converter8/1
  Data Type Conversion/1 -> [above20]  "0.2"
  Compare To Constant1/1 -> Data Type Conversion1/1  "0.9"
  Data Type Conversion1/1 -> [below90]  "0.9"
  PS-Simulink Converter2/1 -> C to Ah/1
  V_ref/1 -> Subsystem/1(V_Ref)  "V_ref"
  PS-Simulink Converter1/1 -> [Batt_V]  "V_batt"
  into SOC/1 -> Compare To Constant1/1, To Workspace17/1, [Batt_SOC], Subsystem/3(soc), Scope/1, Compare To Constant/1  "soc"
  Probe1/1 -> To Workspace18/1  "V_probe"
  Probe2/1 -> To Workspace19/1  "I_probe"
  Subsystem/2(PWM_bottom) -> Simulink-PS Converter9/1
  Compare To Constant/1 -> Data Type Conversion/1  "0.2"
  connections:
  Voltage Sensor Cathode3/RConn2 -- Switch3/LConn1 -- Resistor7/RConn1 -- Solar Cell/RConn1 -- Voltage Sensor/RConn2 -- Solver Configuration1/RConn1 -- Electrical Reference1/LConn1 -- Current Sensor/RConn2
  Simulink-PS Converter5/RConn1 -- Solar Cell/LConn1
  Current Sensor1/LConn1 -- Resistor5/LConn1 -- Switch/LConn1 -- Solar Cell/LConn2 -- Voltage Sensor/LConn1
  Rint_stack1/LConn1 -- Ra_1_stack1/RConn1 -- Ca_1_stack1/RConn1
  Rint_stack1/RConn1 -- Vint_stack1/LConn1
  Cc_2_stack1/LConn1 -- Vint_stack1/RConn1 -- Rc_2_stack1/LConn1
  Voltage Sensor Cathode3/RConn1 -- PS-Simulink Converter9/LConn1
  Current Sensor1/RConn1 -- PS-Simulink Converter4/LConn1
  PS-Simulink Converter5/LConn1 -- Current Sensor/RConn1
  PS-Simulink Converter3/LConn1 -- Voltage Sensor/RConn1
  Simulink-PS Converter1/RConn1 -- Solar Cell1/LConn1
  PS-Simulink Converter7/LConn1 -- Current Sensor2/RConn1
  Voltage Sensor2/LConn1 -- Current Sensor2/LConn1 -- Solar Cell1/LConn2
  Switch1/LConn1 -- Resistor4/LConn1 -- Current Sensor4/RConn2 -- Resistor5/RConn1 -- Switch/RConn2
  Simulink-PS Converter2/RConn1 -- Solar Cell2/LConn1
  Solar Cell2/RConn1 -- Voltage Sensor3/RConn2 -- Resistor6/RConn1 -- Switch2/LConn1 -- Resistor7/LConn1 -- Switch3/RConn2
  Simulink-PS Converter/RConn1 -- Switch3/RConn1
  Simulink-PS Converter6/RConn1 -- Switch/RConn1
  Simulink-PS Converter3/RConn1 -- Switch2/RConn1
  Switch1/RConn1 -- Simulink-PS Converter4/RConn1
  PS-Simulink Converter8/LConn1 -- Voltage Sensor2/RConn1
  PS-Simulink Converter10/LConn1 -- Voltage Sensor3/RConn1
  Resistor/LConn1 -- Switch4/LConn1
  PS-Simulink Converter6/LConn1 -- Current Sensor4/RConn1
  Voltage Sensor3/LConn1 -- Current Sensor4/LConn1 -- Solar Cell2/LConn2
  Switch2/RConn2 -- Switch11/LConn1 -- Voltage Sensor2/RConn2 -- Solar Cell1/RConn1 -- Resistor6/LConn1
  Ca_1_stack1/LConn1 -- Ra_1_stack1/LConn1 -- Bidirectional DC-DC Converter/LConn2 -- Current Sensor1/RConn2 -- Voltage Sensor Cathode3/LConn1
  Rc_2_stack1/RConn1 -- Current Sensor/LConn1 -- Cc_2_stack1/RConn1
  Simulink-PS Converter14/RConn1 -- Switch11/RConn1
  Switch1/RConn2 -- Resistor4/RConn1 -- Switch4/RConn2 -- Current Sensor2/RConn2
  Simulink-PS Converter7/RConn1 -- Switch4/RConn1
  Switch11/RConn2 -- Resistor/RConn1
  Battery1/LConn1 -- Bidirectional DC-DC Converter/RConn1 -- V_out1/LConn1
  Electrical Reference2/LConn1 -- Battery1/RConn1 -- V_out1/RConn2
  V_out1/RConn1 -- PS-Simulink Converter1/LConn1
  PS-Simulink Converter2/LConn1 -- Battery1/LConn2
  Two-Pulse Gate Multiplexer/RConn1 -- Bidirectional DC-DC Converter/LConn1
  Simulink-PS Converter9/RConn1 -- Two-Pulse Gate Multiplexer/LConn2
  Electrical Reference4/LConn1 -- Bidirectional DC-DC Converter/RConn2
  Electrical Reference3/LConn1 -- Bidirectional DC-DC Converter/LConn3
  Two-Pulse Gate Multiplexer/LConn1 -- Simulink-PS Converter8/RConn1

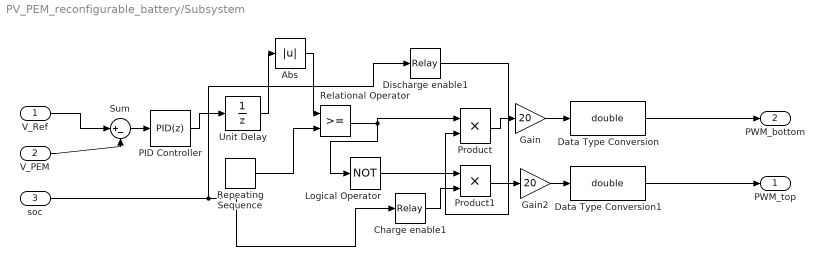
== system  PV_PEM_reconfigurable_battery/Subsystem ==
  V_Ref : Inport
  V_PEM : Inport  Port=2
  soc : Inport  Port=3
  Abs : Abs  SaturateOnIntegerOverflow=off
  Charge enable1 : Relay  OnSwitchValue=0.9  OffSwitchValue=0.85  OnOutputValue=0  OffOutputValue=1
  Data Type Conversion : DataTypeConversion  OutDataTypeStr=double  SaturateOnIntegerOverflow=off  RndMeth=Floor
  Data Type Conversion1 : DataTypeConversion  OutDataTypeStr=double  SaturateOnIntegerOverflow=off  RndMeth=Floor
  Discharge enable1 : Relay  OnSwitchValue=0.25  OffSwitchValue=0.2
  Gain : Gain  Gain=20
  Gain2 : Gain  Gain=20
  Logical Operator : Logic  Operator=NOT  AllPortsSameDT=off  OutDataTypeStr=boolean
  PID Controller : slpidlib/PID Controller  Controller=PID  Form=Parallel  TimeDomain=Discrete-time  UseExternalTs=off  SampleTime=-1  IntegratorMethod=Forward Euler  FilterMethod=Forward Euler  ControllerParametersSource=internal  P=0.05  I=15  UseKiTs=off  D=0  UseExternalDerivativeSource=off  N=100  UseFilter=on  TunerSelectOption=Transfer Function Based (PID Tuner App)  InitialConditionSource=internal  InitialConditionForIntegrator=0.1  InitialConditionForFilter=0.1  DifferentiatorICPrevScaledInput=0  ExternalReset=none  TrackingMode=off  Kt=1  LimitOutput=on  SatLimitsSource=internal  UpperSaturationLimit=0.9  LowerSaturationLimit=0.1  LinearizeAsGain=on  AntiWindupMode=clamping  Kb=1  LimitIntegrator=off  UpperIntegratorSaturationLimit=inf  LowerIntegratorSaturationLimit=-inf  POutMin=[]  POutMax=[]  IOutMin=[]  IOutMax=[]  DOutMin=[]  DOutMax=[]  NOutMin=[]  NOutMax=[]  SumOutMin=[]  SumOutMax=[]  SaturationOutMin=[]  SaturationOutMax=[]  PParamMin=[]  PParamMax=[]  IParamMin=[]  IParamMax=[]  DParamMin=[]  DParamMax=[]  NParamMin=[]  NParamMax=[]  KbParamMin=[]  KbParamMax=[]  KtParamMin=[]  KtParamMax=[]  KbOutMin=[]  KbOutMax=[]  KtOutMin=[]  KtOutMax=[]  IntegratorOutMin=[]  IntegratorOutMax=[]  FilterOutMin=[]  FilterOutMax=[]  SumI1OutMin=[]  SumI1OutMax=[]  SumI2OutMin=[]  SumI2OutMax=[]  SumI3OutMin=[]  SumI3OutMax=[]  SumI4OutMin=[]  SumI4OutMax=[]  SumDOutMin=[]  SumDOutMax=[]  DifferentiatorOutMin=[]  DifferentiatorOutMax=[]  FilterDiffOutCoefMin=[]  FilterDiffOutCoefMax=[]  ReciprocalOutMin=[]  ReciprocalOutMax=[]  SumDenOutMin=[]  SumDenOutMax=[]  SumNumOutMin=[]  SumNumOutMax=[]  DivideOutMin=[]  DivideOutMax=[]  UdiffTsProdOutMin=[]  UdiffTsProdOutMax=[]  NTsProdOutMin=[]  NTsProdOutMax=[]  UintegralTsProdOutMin=[]  UintegralTsProdOutMax=[]  UngainTsProdOutMin=[]  UngainTsProdOutMax=[]  ClampingZeroOutDataTypeStr=Inherit: Inherit via back propagation  ClampingZeroOutMin=[]  ClampingZeroOutMax=[]  FilterDenConstantOutDataTypeStr=Inherit: Inherit via back propagation  FilterDenConstantOutMin=[]  FilterDenConstantOutMax=[]  PCopyOutDataTypeStr=Inherit: Inherit via back propagation  PCopyOutMin=[]  PCopyOutMax=[]  NCopyOutDataTypeStr=Inherit: Inherit via back propagation  NCopyOutMin=[]  NCopyOutMax=[]  IntegratorContinuousStateAttributes=''  IntegratorStateIdentifier=1e-4  IntegratorStateMustResolveToSignalObject=off  IntegratorRTWStateStorageClass=Auto  FilterContinuousStateAttributes=''  FilterStateMustResolveToSignalObject=off  FilterRTWStateStorageClass=Auto  ParallelPVariant=InternalParameters  IdealPVariant=Disabled  IVariant=InternalParameters  DVariant=InternalParameters  IntegratorVariant=Discrete  SatVariant=Enabled  AWVariant=DiscClampingParallel  PCopyVariant=Disabled  TRVariant=Disabled  FdbkBlocksVariant=Forward  IdealPFdbkVariant=Disabled  SatFdbkVariant=Disabled  DerivativeFilterVariant=ForwardEulerFilter  NVariant=InternalParameters  NCopyVariant=Disabled  FilterICVariant=InternalICsFilter  IntegratorICVariant=InternalICs  ExternalResetVariant=Disabled  TRSumVariant=Passthrough  SumFdbkVariant=Disabled  SumVariant=Sum_PID  TsampFilterVariant=InternalTs  TsampNgainVariant=Passthrough  TsampIntegralVariant=Disabled_SignalSpec  ExternalSaturationOutDataTypeStr=Inherit: Same as second input  DerivativeSourceVariant=ErrorSignal  PreIntVariant=InternalPreInt
  Product : Product
  Product1 : Product
  Relational Operator : RelationalOperator  OutDataTypeStr=boolean  RndMeth=Simplest  InputSameDT=off
  Repeating Sequence : simulink/Sources/Repeating Sequence  rep_seq_t=[0, 1e-4]  rep_seq_y=[0, 1]
  Sum : Sum  Inputs=|+-
  Unit Delay : UnitDelay  InitialCondition=0.05  SampleTime=Ts
  PWM_top : Outport  VectorParamsAs1DForOutWhenUnconnected=off
  PWM_bottom : Outport  Port=2  VectorParamsAs1DForOutWhenUnconnected=off
  wires:
  Repeating Sequence/1 -> Relational Operator/2
  Gain/1 -> Data Type Conversion/1
  Gain2/1 -> Data Type Conversion1/1
  PID Controller/1 -> Unit Delay/1
  Relational Operator/1 -> Logical Operator/1, Product/1
  Logical Operator/1 -> Product1/1
  Sum/1 -> PID Controller/1
  V_Ref/1 -> Sum/1
  V_PEM/1 -> Sum/2
  Data Type Conversion1/1 -> PWM_top/1
  Discharge enable1/1 -> Product/2
  Charge enable1/1 -> Product1/2
  Product1/1 -> Gain2/1
  Product/1 -> Gain/1
  soc/1 -> Charge enable1/1, Discharge enable1/1
  Data Type Conversion/1 -> PWM_bottom/1
  Abs/1 -> Relational Operator/1
  Unit Delay/1 -> Abs/1

== matlab function  PV_PEM_reconfigurable_battery/Metrics calculations ==
  data: P_PEM input; I input; Vint input; R1 input; R2 input; Rint input; eta_electrical output; eta_chemical output; eta_F output; n_dot output; m_dot output; P_chemical output; P_loss output; yield output; N input

function [eta_electrical, eta_chemical, eta_F,n_dot, m_dot,P_chemical, P_loss, yield]   = pem_eff( P_PEM, I,Vint, R1, R2, Rint, N)

Rsum = R1 + R2 + Rint;
eta_electrical = (I*Vint) / (I*Vint + I^2 * Rsum); % Guilbert et al. = eta electrical = eta_PV_H2

area = 0.005; %[m^2]
i_el = I / area; %current density [A/m^2]
eta_F_percent = 96.5 * exp(0.09 / i_el - 75.5 / i_el^2);  %Yodwong et al.
eta_F = eta_F_percent/100; 
F_constant = 96485.33; %[s*A/mol]

n_dot = eta_F*I*N/(2*F_constant); %[mol/s]

HHV = 286000; %[J/mol]
P_chemical = n_dot * HHV; %[W]

molar_mass = 2.016; %[g/mol]
m_dot = n_dot * molar_mass; % [g/s]
m_dot_kg_h = m_dot * 3.6; %[kg/h]

eta_chemical = P_chemical/P_PEM; 

P_loss = P_PEM - P_chemical; 

yield = m_dot_kg_h/(P_PEM/1000); %[kg/Wh]


end
%Faradaic efficiency = 1 which means that the resulting efficiency and
%hydrogen production is the upper limit
%change it later to variables being saved in a way that they can be used in the function and onl need I input
% eta equation from Guilbert et al.

== matlab function  PV_PEM_reconfigurable_battery/MATLAB Function ==
  settings: updateMethod=DISCRETE  sampleTime=Ts
  data: irr input; THR_97_up input; THR_97_down input; sw_1 output; sw_2 output; sw_disconnect output; THR_75_up input; THR_75_down input; np_override input
function [sw_1, sw_2, sw_disconnect] = Recon_sw(irr, THR_97_up, THR_97_down, THR_75_up, THR_75_down, np_override)
% Recon_sw  Reconfigurable PV string switching logic.
%
%   np_override – Python real-time Np decision fed from a "From Workspace"
%                 block reading Np_py_ts (built before sim() by the MATLAB
%                 pre-computation block).  Value is 5, 6, or 7.
%                 Set to 0 to activate the threshold hysteresis fallback.

    % ── Python real-time override (np_override > 0) ───────────────────────
    if np_override > 0
        switch round(np_override)
            case 7,  sw_1 = 1;  sw_2 = 1;  sw_disconnect = 0;   % Low-G  (12 str equiv)
            case 6,  sw_1 = 1;  sw_2 = 0;  sw_disconnect = 1;   % Mid-G  (10 str equiv)
            case 5,  sw_1 = 0;  sw_2 = 1;  sw_disconnect = 1;   % High-G ( 8 str equiv)
            otherwise, sw_1 = 1;  sw_2 = 1;  sw_disconnect = 0;
        end
        return;                                                   % ← skip state machine
    end

    % ── Fallback: original threshold-based hysteresis logic ───────────────
    persistent np_state
    if isempty(np_state)
        np_state = 12;   % startup: all 12 strings connected (Low-G)
    end

    % ── State transition logic ────────────────────────────────────────────
    switch np_state
        case 12
            if irr >= THR_97_up
                np_state = 10;
            end

        case 10
            if irr >= THR_75_up
                np_state = 8;
            elseif irr <= THR_97_down
                np_state = 12;
            end

        case 8
            if irr <= THR_97_down        % large drop: skip directly to 12
                np_state = 12;
            elseif irr <= THR_75_down    % moderate drop: step to 10
                np_state = 10;
            end
    end

    % ── Output assignment ─────────────────────────────────────────────────
    switch np_state
        case 12,  sw_1 = 1;  sw_2 = 1;  sw_disconnect = 0;
        case 10,  sw_1 = 1;  sw_2 = 0;  sw_disconnect = 1;
        case 8,   sw_1 = 0;  sw_2 = 1;  sw_disconnect = 1;
        otherwise, sw_1 = 1;  sw_2 = 1;  sw_disconnect = 0;
    end
end
